simulink model "ASK"  (R2023b)
settings: Solver=VariableStepAuto  StartTime=0.0  StopTime=50  RelTol=1e-3
libraries: commrandsrc3 x1, dspfdesign x1
settings Model: Creator=HP  LastModifiedBy=HP

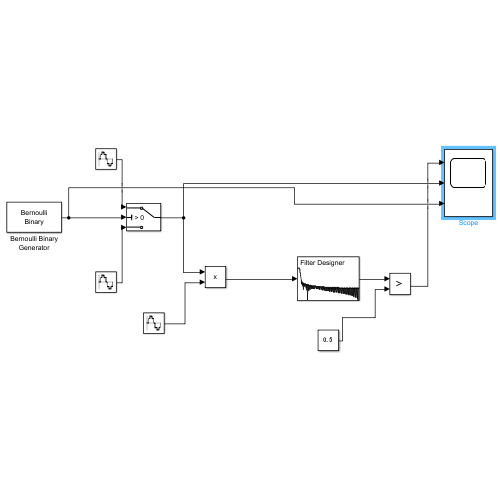
[thumbnail: Simulink's stored preview of the top-level diagram]
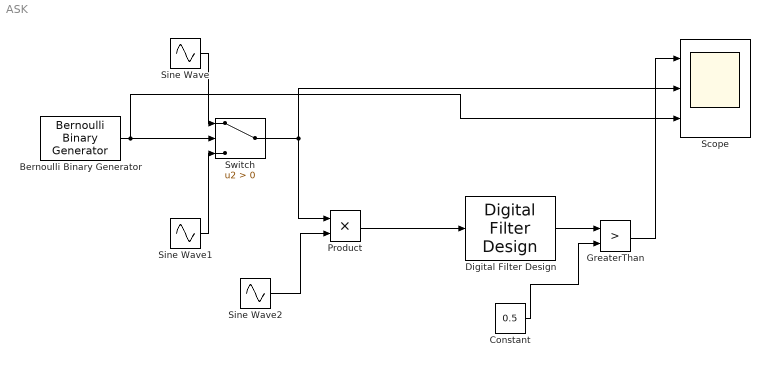
== system ASK ==
  Bernoulli Binary Generator : commrandsrc3/Bernoulli Binary Generator  ProbabilityOfZero=0.5  SeedSource=Auto  Seed=0  SampleTime=1  SamplesPerFrame=1  OutputDataType=double  SimulateUsing=Interpreted execution
  Constant : Constant  Value=0.5
  Digital Filter Design : dspfdesign/Digital Filter Design  mwdsp_browser_bugfix_var=off
  GreaterThan : RelationalOperator  Operator=>  OutDataTypeStr=boolean  RndMeth=Simplest  InputSameDT=off
  Product : Product
  Scope : Scope  NumInputPorts=3
  Sine Wave : Sin  Amplitude=2  Frequency=4*pi  SampleTime=0.01
  Sine Wave1 : Sin  Amplitude=0.5  Frequency=4*pi  SampleTime=0.01
  Sine Wave2 : Sin  Frequency=4*pi  SampleTime=0.01
  Switch : Switch  Criteria=u2 > Threshold  SaturateOnIntegerOverflow=off  InputSameDT=off
  wires:
  Constant/1 -> GreaterThan/2
  Sine Wave/1 -> Switch/1
  Sine Wave1/1 -> Switch/3
  Switch/1 -> Product/1, Scope/2
  Sine Wave2/1 -> Product/2
  Product/1 -> Digital Filter Design/1
  Digital Filter Design/1 -> GreaterThan/1
  GreaterThan/1 -> Scope/1
  Bernoulli Binary Generator/1 -> Scope/3, Switch/2
